simulink model "lab3_kalman"  (R2023b)
settings: Solver=ode45  StartTime=0.0  StopTime=120  RelTol=1e-3
settings Model: Creator=Daniela  LastModifiedBy=Daniela

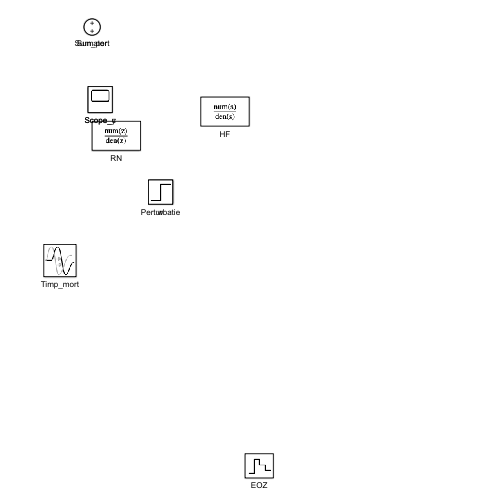
[thumbnail: Simulink's stored preview of the top-level diagram]
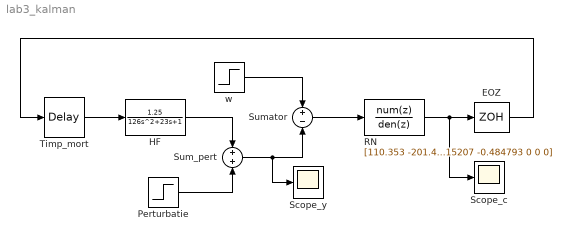
== system lab3_kalman ==
  EOZ : ZeroOrderHold
  HF : TransferFcn  Numerator=1.25  Denominator=[126 23 1]
  Perturbatie : Step  Time=0  After=0  SampleTime=0
  RN : DiscreteTransferFcn  Numerator=[110.353 -201.493 91.9405]  Denominator=[1 -0.515207 -0.484793 0 0 0]  SampleTime=1
  Scope_c : Scope
  Scope_y : Scope
  Sum_pert : Sum
  Sumator : Sum  Inputs=+-
  Timp_mort : TransportDelay  DelayTime=3
  w : Step  Time=0  SampleTime=0
  wires:
  Sum_pert/1 -> Sumator/2, Scope_y/1
  Perturbatie/1 -> Sum_pert/2
  HF/1 -> Sum_pert/1
  Timp_mort/1 -> HF/1
  EOZ/1 -> Timp_mort/1
  RN/1 -> EOZ/1, Scope_c/1
  Sumator/1 -> RN/1
  w/1 -> Sumator/1
